simulink model "TRN_current"  (Simulink 6.2)
settings: Solver=ode45  SolverMode=SingleTasking  StartTime=0  StopTime=6  MaxStep=0.1  RelTol=1e-3  AbsTol=1e-3
libraries: simulink x1
(part 2 of 3)

== system TRN_current/Basal Ganglia/Striatum(D1)/chan1 ==
  note: Dopamine
      | modulation
  dopamine : Inport  Orientation=down  Port=1  PortDimensions=1  LatchInput=off
  cortex : Inport  Orientation=down  Port=2  LatchInput=off
  salience : Inport  Orientation=down  Port=3  LatchInput=off
  Constant : Constant  Orientation=down
  Product : Product  Orientation=down  SaturateOnIntegerOverflow=on  RndMeth=Zero  InputSameDT=on
  Sum : Sum  Orientation=down  SaturateOnIntegerOverflow=on  InputSameDT=on
  Sum1 : Sum  Orientation=down  SaturateOnIntegerOverflow=on  InputSameDT=on
  leaky integration : Subsystem  Orientation=down
  piecewise lin. : S-Function  Orientation=down  FunctionName=Mpieclin  Parameters=slope,thresh
  weight : Gain  Orientation=down  Gain=W_ctx  SaturateOnIntegerOverflow=on
  weight1 : Gain  Orientation=down  Gain=W_sal  SaturateOnIntegerOverflow=on
  out : Outport  Orientation=down  InitialOutput=0
  wires:
  Product/1 -> leaky integration/1(Inport)
  Constant/1 -> Sum/1
  piecewise lin./1 -> out/1
  leaky integration/1(Outport) -> piecewise lin./1
  dopamine/1 -> Sum/2
  Sum/1 -> Product/1
  cortex/1 -> weight/1
  salience/1 -> weight1/1
  weight/1 -> Sum1/1
  weight1/1 -> Sum1/2
  Sum1/1 -> Product/2

== system TRN_current/Basal Ganglia/Striatum(D1)/chan2 ==
  note: Dopamine
      | modulation
  dopamine : Inport  Orientation=down  Port=1  PortDimensions=1  LatchInput=off
  cortex : Inport  Orientation=down  Port=2  LatchInput=off
  salience : Inport  Orientation=down  Port=3  LatchInput=off
  Constant : Constant  Orientation=down
  Product : Product  Orientation=down  SaturateOnIntegerOverflow=on  RndMeth=Zero  InputSameDT=on
  Sum : Sum  Orientation=down  SaturateOnIntegerOverflow=on  InputSameDT=on
  Sum1 : Sum  Orientation=down  SaturateOnIntegerOverflow=on  InputSameDT=on
  leaky integration : Subsystem  Orientation=down
  piecewise lin. : S-Function  Orientation=down  FunctionName=Mpieclin  Parameters=slope,thresh
  weight : Gain  Orientation=down  Gain=W_ctx  SaturateOnIntegerOverflow=on
  weight1 : Gain  Orientation=down  Gain=W_sal  SaturateOnIntegerOverflow=on
  out : Outport  Orientation=down  InitialOutput=0
  wires:
  Sum1/1 -> Product/2
  weight1/1 -> Sum1/2
  weight/1 -> Sum1/1
  salience/1 -> weight1/1
  cortex/1 -> weight/1
  Sum/1 -> Product/1
  dopamine/1 -> Sum/2
  leaky integration/1(Outport) -> piecewise lin./1
  piecewise lin./1 -> out/1
  Constant/1 -> Sum/1
  Product/1 -> leaky integration/1(Inport)

== system TRN_current/Basal Ganglia/Striatum(D1)/chan3 ==
  note: Dopamine
      | modulation
  dopamine : Inport  Orientation=down  Port=1  PortDimensions=1  LatchInput=off
  cortex : Inport  Orientation=down  Port=2  LatchInput=off
  salience : Inport  Orientation=down  Port=3  LatchInput=off
  Constant : Constant  Orientation=down
  Product : Product  Orientation=down  SaturateOnIntegerOverflow=on  RndMeth=Zero  InputSameDT=on
  Sum : Sum  Orientation=down  SaturateOnIntegerOverflow=on  InputSameDT=on
  Sum1 : Sum  Orientation=down  SaturateOnIntegerOverflow=on  InputSameDT=on
  leaky integration : Subsystem  Orientation=down
  piecewise lin. : S-Function  Orientation=down  FunctionName=Mpieclin  Parameters=slope,thresh
  weight : Gain  Orientation=down  Gain=W_ctx  SaturateOnIntegerOverflow=on
  weight1 : Gain  Orientation=down  Gain=W_sal  SaturateOnIntegerOverflow=on
  out : Outport  Orientation=down  InitialOutput=0
  wires:
  Product/1 -> leaky integration/1(Inport)
  Constant/1 -> Sum/1
  piecewise lin./1 -> out/1
  leaky integration/1(Outport) -> piecewise lin./1
  dopamine/1 -> Sum/2
  Sum/1 -> Product/1
  cortex/1 -> weight/1
  salience/1 -> weight1/1
  weight/1 -> Sum1/1
  weight1/1 -> Sum1/2
  Sum1/1 -> Product/2

== system TRN_current/Basal Ganglia/Striatum(D1)/chan4 ==
  note: Dopamine
      | modulation
  dopamine : Inport  Orientation=down  Port=1  PortDimensions=1  LatchInput=off
  cortex : Inport  Orientation=down  Port=2  LatchInput=off
  salience : Inport  Orientation=down  Port=3  LatchInput=off
  Constant : Constant  Orientation=down
  Product : Product  Orientation=down  SaturateOnIntegerOverflow=on  RndMeth=Zero  InputSameDT=on
  Sum : Sum  Orientation=down  SaturateOnIntegerOverflow=on  InputSameDT=on
  Sum1 : Sum  Orientation=down  SaturateOnIntegerOverflow=on  InputSameDT=on
  leaky integration : Subsystem  Orientation=down
  piecewise lin. : S-Function  Orientation=down  FunctionName=Mpieclin  Parameters=slope,thresh
  weight : Gain  Orientation=down  Gain=W_ctx  SaturateOnIntegerOverflow=on
  weight1 : Gain  Orientation=down  Gain=W_sal  SaturateOnIntegerOverflow=on
  out : Outport  Orientation=down  InitialOutput=0
  wires:
  Sum1/1 -> Product/2
  weight1/1 -> Sum1/2
  weight/1 -> Sum1/1
  salience/1 -> weight1/1
  cortex/1 -> weight/1
  Sum/1 -> Product/1
  dopamine/1 -> Sum/2
  leaky integration/1(Outport) -> piecewise lin./1
  piecewise lin./1 -> out/1
  Constant/1 -> Sum/1
  Product/1 -> leaky integration/1(Inport)

== system TRN_current/Basal Ganglia/Striatum(D1)/chan5 ==
  note: Dopamine
      | modulation
  dopamine : Inport  Orientation=down  Port=1  PortDimensions=1  LatchInput=off
  cortex : Inport  Orientation=down  Port=2  LatchInput=off
  salience : Inport  Orientation=down  Port=3  LatchInput=off
  Constant : Constant  Orientation=down
  Product : Product  Orientation=down  SaturateOnIntegerOverflow=on  RndMeth=Zero  InputSameDT=on
  Sum : Sum  Orientation=down  SaturateOnIntegerOverflow=on  InputSameDT=on
  Sum1 : Sum  Orientation=down  SaturateOnIntegerOverflow=on  InputSameDT=on
  leaky integration : Subsystem  Orientation=down
  piecewise lin. : S-Function  Orientation=down  FunctionName=Mpieclin  Parameters=slope,thresh
  weight : Gain  Orientation=down  Gain=W_ctx  SaturateOnIntegerOverflow=on
  weight1 : Gain  Orientation=down  Gain=W_sal  SaturateOnIntegerOverflow=on
  out : Outport  Orientation=down  InitialOutput=0
  wires:
  Product/1 -> leaky integration/1(Inport)
  Constant/1 -> Sum/1
  piecewise lin./1 -> out/1
  leaky integration/1(Outport) -> piecewise lin./1
  dopamine/1 -> Sum/2
  Sum/1 -> Product/1
  cortex/1 -> weight/1
  salience/1 -> weight1/1
  weight/1 -> Sum1/1
  weight1/1 -> Sum1/2
  Sum1/1 -> Product/2

== system TRN_current/Basal Ganglia/Striatum(D1)/chan6 ==
  note: Dopamine
      | modulation
  dopamine : Inport  Orientation=down  Port=1  PortDimensions=1  LatchInput=off
  cortex : Inport  Orientation=down  Port=2  LatchInput=off
  salience : Inport  Orientation=down  Port=3  LatchInput=off
  Constant : Constant  Orientation=down
  Product : Product  Orientation=down  SaturateOnIntegerOverflow=on  RndMeth=Zero  InputSameDT=on
  Sum : Sum  Orientation=down  SaturateOnIntegerOverflow=on  InputSameDT=on
  Sum1 : Sum  Orientation=down  SaturateOnIntegerOverflow=on  InputSameDT=on
  leaky integration : Subsystem  Orientation=down
  piecewise lin. : S-Function  Orientation=down  FunctionName=Mpieclin  Parameters=slope,thresh
  weight : Gain  Orientation=down  Gain=W_ctx  SaturateOnIntegerOverflow=on
  weight1 : Gain  Orientation=down  Gain=W_sal  SaturateOnIntegerOverflow=on
  out : Outport  Orientation=down  InitialOutput=0
  wires:
  Sum1/1 -> Product/2
  weight1/1 -> Sum1/2
  weight/1 -> Sum1/1
  salience/1 -> weight1/1
  cortex/1 -> weight/1
  Sum/1 -> Product/1
  dopamine/1 -> Sum/2
  leaky integration/1(Outport) -> piecewise lin./1
  piecewise lin./1 -> out/1
  Constant/1 -> Sum/1
  Product/1 -> leaky integration/1(Inport)

== system TRN_current/Basal Ganglia/Striatum(D2)/chan1 ==
  note: Dopamine
      | modulation
  dopamine : Inport  Orientation=down  Port=1  PortDimensions=1  LatchInput=off
  cortex : Inport  Orientation=down  Port=2  LatchInput=off
  salience : Inport  Orientation=down  Port=3  LatchInput=off
  Constant : Constant  Orientation=down
  Product : Product  Orientation=down  SaturateOnIntegerOverflow=on  RndMeth=Zero  InputSameDT=on
  Sum : Sum  Orientation=down  Inputs=+-  SaturateOnIntegerOverflow=on  InputSameDT=on
  Sum1 : Sum  Orientation=down  SaturateOnIntegerOverflow=on  InputSameDT=on
  leaky integration : Subsystem  Orientation=down
  piecewise lin. : S-Function  Orientation=down  FunctionName=Mpieclin  Parameters=slope,thresh
  weight : Gain  Orientation=down  Gain=W_ctx  SaturateOnIntegerOverflow=on
  weight1 : Gain  Orientation=down  Gain=W_sal  SaturateOnIntegerOverflow=on
  out : Outport  Orientation=down  InitialOutput=0
  wires:
  Sum1/1 -> Product/2
  weight1/1 -> Sum1/2
  weight/1 -> Sum1/1
  salience/1 -> weight1/1
  cortex/1 -> weight/1
  Sum/1 -> Product/1
  dopamine/1 -> Sum/2
  leaky integration/1(Outport) -> piecewise lin./1
  piecewise lin./1 -> out/1
  Constant/1 -> Sum/1
  Product/1 -> leaky integration/1(Inport)

== system TRN_current/Basal Ganglia/Striatum(D2)/chan2 ==
  note: Dopamine
      | modulation
  dopamine : Inport  Orientation=down  Port=1  PortDimensions=1  LatchInput=off
  cortex : Inport  Orientation=down  Port=2  LatchInput=off
  salience : Inport  Orientation=down  Port=3  LatchInput=off
  Constant : Constant  Orientation=down
  Product : Product  Orientation=down  SaturateOnIntegerOverflow=on  RndMeth=Zero  InputSameDT=on
  Sum : Sum  Orientation=down  Inputs=+-  SaturateOnIntegerOverflow=on  InputSameDT=on
  Sum1 : Sum  Orientation=down  SaturateOnIntegerOverflow=on  InputSameDT=on
  leaky integration : Subsystem  Orientation=down
  piecewise lin. : S-Function  Orientation=down  FunctionName=Mpieclin  Parameters=slope,thresh
  weight : Gain  Orientation=down  Gain=W_ctx  SaturateOnIntegerOverflow=on
  weight1 : Gain  Orientation=down  Gain=W_sal  SaturateOnIntegerOverflow=on
  out : Outport  Orientation=down  InitialOutput=0
  wires:
  Product/1 -> leaky integration/1(Inport)
  Constant/1 -> Sum/1
  piecewise lin./1 -> out/1
  leaky integration/1(Outport) -> piecewise lin./1
  dopamine/1 -> Sum/2
  Sum/1 -> Product/1
  cortex/1 -> weight/1
  salience/1 -> weight1/1
  weight/1 -> Sum1/1
  weight1/1 -> Sum1/2
  Sum1/1 -> Product/2

== system TRN_current/Basal Ganglia/Striatum(D2)/chan3 ==
  note: Dopamine
      | modulation
  dopamine : Inport  Orientation=down  Port=1  PortDimensions=1  LatchInput=off
  cortex : Inport  Orientation=down  Port=2  LatchInput=off
  salience : Inport  Orientation=down  Port=3  LatchInput=off
  Constant : Constant  Orientation=down
  Product : Product  Orientation=down  SaturateOnIntegerOverflow=on  RndMeth=Zero  InputSameDT=on
  Sum : Sum  Orientation=down  Inputs=+-  SaturateOnIntegerOverflow=on  InputSameDT=on
  Sum1 : Sum  Orientation=down  SaturateOnIntegerOverflow=on  InputSameDT=on
  leaky integration : Subsystem  Orientation=down
  piecewise lin. : S-Function  Orientation=down  FunctionName=Mpieclin  Parameters=slope,thresh
  weight : Gain  Orientation=down  Gain=W_ctx  SaturateOnIntegerOverflow=on
  weight1 : Gain  Orientation=down  Gain=W_sal  SaturateOnIntegerOverflow=on
  out : Outport  Orientation=down  InitialOutput=0
  wires:
  Sum1/1 -> Product/2
  weight1/1 -> Sum1/2
  weight/1 -> Sum1/1
  salience/1 -> weight1/1
  cortex/1 -> weight/1
  Sum/1 -> Product/1
  dopamine/1 -> Sum/2
  leaky integration/1(Outport) -> piecewise lin./1
  piecewise lin./1 -> out/1
  Constant/1 -> Sum/1
  Product/1 -> leaky integration/1(Inport)

== system TRN_current/Basal Ganglia/Striatum(D2)/chan4 ==
  note: Dopamine
      | modulation
  dopamine : Inport  Orientation=down  Port=1  PortDimensions=1  LatchInput=off
  cortex : Inport  Orientation=down  Port=2  LatchInput=off
  salience : Inport  Orientation=down  Port=3  LatchInput=off
  Constant : Constant  Orientation=down
  Product : Product  Orientation=down  SaturateOnIntegerOverflow=on  RndMeth=Zero  InputSameDT=on
  Sum : Sum  Orientation=down  Inputs=+-  SaturateOnIntegerOverflow=on  InputSameDT=on
  Sum1 : Sum  Orientation=down  SaturateOnIntegerOverflow=on  InputSameDT=on
  leaky integration : Subsystem  Orientation=down
  piecewise lin. : S-Function  Orientation=down  FunctionName=Mpieclin  Parameters=slope,thresh
  weight : Gain  Orientation=down  Gain=W_ctx  SaturateOnIntegerOverflow=on
  weight1 : Gain  Orientation=down  Gain=W_sal  SaturateOnIntegerOverflow=on
  out : Outport  Orientation=down  InitialOutput=0
  wires:
  Product/1 -> leaky integration/1(Inport)
  Constant/1 -> Sum/1
  piecewise lin./1 -> out/1
  leaky integration/1(Outport) -> piecewise lin./1
  dopamine/1 -> Sum/2
  Sum/1 -> Product/1
  cortex/1 -> weight/1
  salience/1 -> weight1/1
  weight/1 -> Sum1/1
  weight1/1 -> Sum1/2
  Sum1/1 -> Product/2

== system TRN_current/Basal Ganglia/Striatum(D2)/chan5 ==
  note: Dopamine
      | modulation
  dopamine : Inport  Orientation=down  Port=1  PortDimensions=1  LatchInput=off
  cortex : Inport  Orientation=down  Port=2  LatchInput=off
  salience : Inport  Orientation=down  Port=3  LatchInput=off
  Constant : Constant  Orientation=down
  Product : Product  Orientation=down  SaturateOnIntegerOverflow=on  RndMeth=Zero  InputSameDT=on
  Sum : Sum  Orientation=down  Inputs=+-  SaturateOnIntegerOverflow=on  InputSameDT=on
  Sum1 : Sum  Orientation=down  SaturateOnIntegerOverflow=on  InputSameDT=on
  leaky integration : Subsystem  Orientation=down
  piecewise lin. : S-Function  Orientation=down  FunctionName=Mpieclin  Parameters=slope,thresh
  weight : Gain  Orientation=down  Gain=W_ctx  SaturateOnIntegerOverflow=on
  weight1 : Gain  Orientation=down  Gain=W_sal  SaturateOnIntegerOverflow=on
  out : Outport  Orientation=down  InitialOutput=0
  wires:
  Sum1/1 -> Product/2
  weight1/1 -> Sum1/2
  weight/1 -> Sum1/1
  salience/1 -> weight1/1
  cortex/1 -> weight/1
  Sum/1 -> Product/1
  dopamine/1 -> Sum/2
  leaky integration/1(Outport) -> piecewise lin./1
  piecewise lin./1 -> out/1
  Constant/1 -> Sum/1
  Product/1 -> leaky integration/1(Inport)

== system TRN_current/Basal Ganglia/Striatum(D2)/chan6 ==
  note: Dopamine
      | modulation
  dopamine : Inport  Orientation=down  Port=1  PortDimensions=1  LatchInput=off
  cortex : Inport  Orientation=down  Port=2  LatchInput=off
  salience : Inport  Orientation=down  Port=3  LatchInput=off
  Constant : Constant  Orientation=down
  Product : Product  Orientation=down  SaturateOnIntegerOverflow=on  RndMeth=Zero  InputSameDT=on
  Sum : Sum  Orientation=down  Inputs=+-  SaturateOnIntegerOverflow=on  InputSameDT=on
  Sum1 : Sum  Orientation=down  SaturateOnIntegerOverflow=on  InputSameDT=on
  leaky integration : Subsystem  Orientation=down
  piecewise lin. : S-Function  Orientation=down  FunctionName=Mpieclin  Parameters=slope,thresh
  weight : Gain  Orientation=down  Gain=W_ctx  SaturateOnIntegerOverflow=on
  weight1 : Gain  Orientation=down  Gain=W_sal  SaturateOnIntegerOverflow=on
  out : Outport  Orientation=down  InitialOutput=0
  wires:
  Product/1 -> leaky integration/1(Inport)
  Constant/1 -> Sum/1
  piecewise lin./1 -> out/1
  leaky integration/1(Outport) -> piecewise lin./1
  dopamine/1 -> Sum/2
  Sum/1 -> Product/1
  cortex/1 -> weight/1
  salience/1 -> weight1/1
  weight/1 -> Sum1/1
  weight1/1 -> Sum1/2
  Sum1/1 -> Product/2

== system TRN_current/Motor  Cortex/chan1/leaky integration ==
  Inport : Inport  Port=1  PortDimensions=1  LatchInput=off
  Gain : Gain  Gain=A_rate  SaturateOnIntegerOverflow=on
  Integrator : Integrator
  decay const : Gain  Orientation=left  Gain=-A_rate  SaturateOnIntegerOverflow=on
  sum : Sum  SaturateOnIntegerOverflow=on  InputSameDT=on
  Outport : Outport  InitialOutput=0
  wires:
  decay const/1 -> sum/2
  sum/1 -> Integrator/1
  Integrator/1 -> decay const/1, Outport/1
  Inport/1 -> Gain/1
  Gain/1 -> sum/1

== system TRN_current/Motor  Cortex/chan2/leaky integration ==
  Inport : Inport  Port=1  PortDimensions=1  LatchInput=off
  Gain : Gain  Gain=A_rate  SaturateOnIntegerOverflow=on
  Integrator : Integrator
  decay const : Gain  Orientation=left  Gain=-A_rate  SaturateOnIntegerOverflow=on
  sum : Sum  SaturateOnIntegerOverflow=on  InputSameDT=on
  Outport : Outport  InitialOutput=0
  wires:
  Gain/1 -> sum/1
  Inport/1 -> Gain/1
  Integrator/1 -> Outport/1, decay const/1
  sum/1 -> Integrator/1
  decay const/1 -> sum/2

== system TRN_current/Motor  Cortex/chan3/leaky integration ==
  Inport : Inport  Port=1  PortDimensions=1  LatchInput=off
  Gain : Gain  Gain=A_rate  SaturateOnIntegerOverflow=on
  Integrator : Integrator
  decay const : Gain  Orientation=left  Gain=-A_rate  SaturateOnIntegerOverflow=on
  sum : Sum  SaturateOnIntegerOverflow=on  InputSameDT=on
  Outport : Outport  InitialOutput=0
  wires:
  decay const/1 -> sum/2
  sum/1 -> Integrator/1
  Integrator/1 -> decay const/1, Outport/1
  Inport/1 -> Gain/1
  Gain/1 -> sum/1

== system TRN_current/Motor  Cortex/chan4/leaky integration ==
  Inport : Inport  Port=1  PortDimensions=1  LatchInput=off
  Gain : Gain  Gain=A_rate  SaturateOnIntegerOverflow=on
  Integrator : Integrator
  decay const : Gain  Orientation=left  Gain=-A_rate  SaturateOnIntegerOverflow=on
  sum : Sum  SaturateOnIntegerOverflow=on  InputSameDT=on
  Outport : Outport  InitialOutput=0
  wires:
  Gain/1 -> sum/1
  Inport/1 -> Gain/1
  Integrator/1 -> Outport/1, decay const/1
  sum/1 -> Integrator/1
  decay const/1 -> sum/2

== system TRN_current/Motor  Cortex/chan5/leaky integration ==
  Inport : Inport  Port=1  PortDimensions=1  LatchInput=off
  Gain : Gain  Gain=A_rate  SaturateOnIntegerOverflow=on
  Integrator : Integrator
  decay const : Gain  Orientation=left  Gain=-A_rate  SaturateOnIntegerOverflow=on
  sum : Sum  SaturateOnIntegerOverflow=on  InputSameDT=on
  Outport : Outport  InitialOutput=0
  wires:
  decay const/1 -> sum/2
  sum/1 -> Integrator/1
  Integrator/1 -> decay const/1, Outport/1
  Inport/1 -> Gain/1
  Gain/1 -> sum/1

== system TRN_current/Motor  Cortex/chan6/leaky integration ==
  Inport : Inport  Port=1  PortDimensions=1  LatchInput=off
  Gain : Gain  Gain=A_rate  SaturateOnIntegerOverflow=on
  Integrator : Integrator
  decay const : Gain  Orientation=left  Gain=-A_rate  SaturateOnIntegerOverflow=on
  sum : Sum  SaturateOnIntegerOverflow=on  InputSameDT=on
  Outport : Outport  InitialOutput=0
  wires:
  Gain/1 -> sum/1
  Inport/1 -> Gain/1
  Integrator/1 -> Outport/1, decay const/1
  sum/1 -> Integrator/1
  decay const/1 -> sum/2

== system TRN_current/TRN/chan1/leaky integration ==
  Inport : Inport  Port=1  PortDimensions=1  LatchInput=off
  Gain : Gain  Gain=A_rate  SaturateOnIntegerOverflow=on
  Integrator : Integrator
  decay const : Gain  Orientation=left  Gain=-A_rate  SaturateOnIntegerOverflow=on
  sum : Sum  SaturateOnIntegerOverflow=on  InputSameDT=on
  Outport : Outport  InitialOutput=0
  wires:
  decay const/1 -> sum/2
  sum/1 -> Integrator/1
  Integrator/1 -> decay const/1, Outport/1
  Inport/1 -> Gain/1
  Gain/1 -> sum/1

== system TRN_current/TRN/chan2/leaky integration ==
  Inport : Inport  Port=1  PortDimensions=1  LatchInput=off
  Gain : Gain  Gain=A_rate  SaturateOnIntegerOverflow=on
  Integrator : Integrator
  decay const : Gain  Orientation=left  Gain=-A_rate  SaturateOnIntegerOverflow=on
  sum : Sum  SaturateOnIntegerOverflow=on  InputSameDT=on
  Outport : Outport  InitialOutput=0
  wires:
  Gain/1 -> sum/1
  Inport/1 -> Gain/1
  Integrator/1 -> Outport/1, decay const/1
  sum/1 -> Integrator/1
  decay const/1 -> sum/2

== system TRN_current/TRN/chan3/leaky integration ==
  Inport : Inport  Port=1  PortDimensions=1  LatchInput=off
  Gain : Gain  Gain=A_rate  SaturateOnIntegerOverflow=on
  Integrator : Integrator
  decay const : Gain  Orientation=left  Gain=-A_rate  SaturateOnIntegerOverflow=on
  sum : Sum  SaturateOnIntegerOverflow=on  InputSameDT=on
  Outport : Outport  InitialOutput=0
  wires:
  decay const/1 -> sum/2
  sum/1 -> Integrator/1
  Integrator/1 -> decay const/1, Outport/1
  Inport/1 -> Gain/1
  Gain/1 -> sum/1

== system TRN_current/TRN/chan4/leaky integration ==
  Inport : Inport  Port=1  PortDimensions=1  LatchInput=off
  Gain : Gain  Gain=A_rate  SaturateOnIntegerOverflow=on
  Integrator : Integrator
  decay const : Gain  Orientation=left  Gain=-A_rate  SaturateOnIntegerOverflow=on
  sum : Sum  SaturateOnIntegerOverflow=on  InputSameDT=on
  Outport : Outport  InitialOutput=0
  wires:
  Gain/1 -> sum/1
  Inport/1 -> Gain/1
  Integrator/1 -> Outport/1, decay const/1
  sum/1 -> Integrator/1
  decay const/1 -> sum/2

== system TRN_current/TRN/chan5/leaky integration ==
  Inport : Inport  Port=1  PortDimensions=1  LatchInput=off
  Gain : Gain  Gain=A_rate  SaturateOnIntegerOverflow=on
  Integrator : Integrator
  decay const : Gain  Orientation=left  Gain=-A_rate  SaturateOnIntegerOverflow=on
  sum : Sum  SaturateOnIntegerOverflow=on  InputSameDT=on
  Outport : Outport  InitialOutput=0
  wires:
  decay const/1 -> sum/2
  sum/1 -> Integrator/1
  Integrator/1 -> decay const/1, Outport/1
  Inport/1 -> Gain/1
  Gain/1 -> sum/1

== system TRN_current/TRN/chan6/leaky integration ==
  Inport : Inport  Port=1  PortDimensions=1  LatchInput=off
  Gain : Gain  Gain=A_rate  SaturateOnIntegerOverflow=on
  Integrator : Integrator
  decay const : Gain  Orientation=left  Gain=-A_rate  SaturateOnIntegerOverflow=on
  sum : Sum  SaturateOnIntegerOverflow=on  InputSameDT=on
  Outport : Outport  InitialOutput=0
  wires:
  Gain/1 -> sum/1
  Inport/1 -> Gain/1
  Integrator/1 -> Outport/1, decay const/1
  sum/1 -> Integrator/1
  decay const/1 -> sum/2

== system TRN_current/Ventrolateral Thalamus/chan1/leaky integration ==
  Inport : Inport  Port=1  PortDimensions=1  LatchInput=off
  Gain : Gain  Gain=A_rate  SaturateOnIntegerOverflow=on
  Integrator : Integrator
  decay const : Gain  Orientation=left  Gain=-A_rate  SaturateOnIntegerOverflow=on
  sum : Sum  SaturateOnIntegerOverflow=on  InputSameDT=on
  Outport : Outport  InitialOutput=0
  wires:
  decay const/1 -> sum/2
  sum/1 -> Integrator/1
  Integrator/1 -> decay const/1, Outport/1
  Inport/1 -> Gain/1
  Gain/1 -> sum/1

== system TRN_current/Ventrolateral Thalamus/chan2/leaky integration ==
  Inport : Inport  Port=1  PortDimensions=1  LatchInput=off
  Gain : Gain  Gain=A_rate  SaturateOnIntegerOverflow=on
  Integrator : Integrator
  decay const : Gain  Orientation=left  Gain=-A_rate  SaturateOnIntegerOverflow=on
  sum : Sum  SaturateOnIntegerOverflow=on  InputSameDT=on
  Outport : Outport  InitialOutput=0
  wires:
  Gain/1 -> sum/1
  Inport/1 -> Gain/1
  Integrator/1 -> Outport/1, decay const/1
  sum/1 -> Integrator/1
  decay const/1 -> sum/2

== system TRN_current/Ventrolateral Thalamus/chan3/leaky integration ==
  Inport : Inport  Port=1  PortDimensions=1  LatchInput=off
  Gain : Gain  Gain=A_rate  SaturateOnIntegerOverflow=on
  Integrator : Integrator
  decay const : Gain  Orientation=left  Gain=-A_rate  SaturateOnIntegerOverflow=on
  sum : Sum  SaturateOnIntegerOverflow=on  InputSameDT=on
  Outport : Outport  InitialOutput=0
  wires:
  decay const/1 -> sum/2
  sum/1 -> Integrator/1
  Integrator/1 -> decay const/1, Outport/1
  Inport/1 -> Gain/1
  Gain/1 -> sum/1

== system TRN_current/Ventrolateral Thalamus/chan4/leaky integration ==
  Inport : Inport  Port=1  PortDimensions=1  LatchInput=off
  Gain : Gain  Gain=A_rate  SaturateOnIntegerOverflow=on
  Integrator : Integrator
  decay const : Gain  Orientation=left  Gain=-A_rate  SaturateOnIntegerOverflow=on
  sum : Sum  SaturateOnIntegerOverflow=on  InputSameDT=on
  Outport : Outport  InitialOutput=0
  wires:
  Gain/1 -> sum/1
  Inport/1 -> Gain/1
  Integrator/1 -> Outport/1, decay const/1
  sum/1 -> Integrator/1
  decay const/1 -> sum/2

== system TRN_current/Ventrolateral Thalamus/chan5/leaky integration ==
  Inport : Inport  Port=1  PortDimensions=1  LatchInput=off
  Gain : Gain  Gain=A_rate  SaturateOnIntegerOverflow=on
  Integrator : Integrator
  decay const : Gain  Orientation=left  Gain=-A_rate  SaturateOnIntegerOverflow=on
  sum : Sum  SaturateOnIntegerOverflow=on  InputSameDT=on
  Outport : Outport  InitialOutput=0
  wires:
  decay const/1 -> sum/2
  sum/1 -> Integrator/1
  Integrator/1 -> decay const/1, Outport/1
  Inport/1 -> Gain/1
  Gain/1 -> sum/1

== system TRN_current/Ventrolateral Thalamus/chan6/leaky integration ==
  Inport : Inport  Port=1  PortDimensions=1  LatchInput=off
  Gain : Gain  Gain=A_rate  SaturateOnIntegerOverflow=on
  Integrator : Integrator
  decay const : Gain  Orientation=left  Gain=-A_rate  SaturateOnIntegerOverflow=on
  sum : Sum  SaturateOnIntegerOverflow=on  InputSameDT=on
  Outport : Outport  InitialOutput=0
  wires:
  Gain/1 -> sum/1
  Inport/1 -> Gain/1
  Integrator/1 -> Outport/1, decay const/1
  sum/1 -> Integrator/1
  decay const/1 -> sum/2

== system TRN_current/Basal Ganglia/GPe/2 input channel/input summation ==
  x1 : Inport  Port=1  LatchInput=off
  x2 : Inport  Port=2  LatchInput=off
  Sum : Sum  SaturateOnIntegerOverflow=on  InputSameDT=on
  W1 : Gain  Gain=W_str  SaturateOnIntegerOverflow=on
  W2 : Gain  Gain=W_STN  SaturateOnIntegerOverflow=on
  out_1 : Outport  InitialOutput=0
  wires:
  W2/1 -> Sum/2
  W1/1 -> Sum/1
  x2/1 -> W2/1
  x1/1 -> W1/1
  Sum/1 -> out_1/1

== system TRN_current/Basal Ganglia/GPe/2 input channel/leaky integration ==
  Inport : Inport  Port=1  LatchInput=off
  Gain : Gain  Gain=A_rate  SaturateOnIntegerOverflow=on
  Integrator : Integrator
  decay const : Gain  Orientation=left  Gain=-A_rate  SaturateOnIntegerOverflow=on
  sum : Sum  SaturateOnIntegerOverflow=on  InputSameDT=on
  Outport : Outport  InitialOutput=0
  wires:
  Gain/1 -> sum/1
  Inport/1 -> Gain/1
  Integrator/1 -> decay const/1, Outport/1
  sum/1 -> Integrator/1
  decay const/1 -> sum/2

== system TRN_current/Basal Ganglia/GPe/2 input channel1/input summation ==
  x1 : Inport  Port=1  LatchInput=off
  x2 : Inport  Port=2  LatchInput=off
  Sum : Sum  SaturateOnIntegerOverflow=on  InputSameDT=on
  W1 : Gain  Gain=W_str  SaturateOnIntegerOverflow=on
  W2 : Gain  Gain=W_STN  SaturateOnIntegerOverflow=on
  out_1 : Outport  InitialOutput=0
  wires:
  Sum/1 -> out_1/1
  x1/1 -> W1/1
  x2/1 -> W2/1
  W1/1 -> Sum/1
  W2/1 -> Sum/2

== system TRN_current/Basal Ganglia/GPe/2 input channel1/leaky integration ==
  Inport : Inport  Port=1  LatchInput=off
  Gain : Gain  Gain=A_rate  SaturateOnIntegerOverflow=on
  Integrator : Integrator
  decay const : Gain  Orientation=left  Gain=-A_rate  SaturateOnIntegerOverflow=on
  sum : Sum  SaturateOnIntegerOverflow=on  InputSameDT=on
  Outport : Outport  InitialOutput=0
  wires:
  decay const/1 -> sum/2
  sum/1 -> Integrator/1
  Integrator/1 -> Outport/1, decay const/1
  Inport/1 -> Gain/1
  Gain/1 -> sum/1

== system TRN_current/Basal Ganglia/GPe/2 input channel2/input summation ==
  x1 : Inport  Port=1  LatchInput=off
  x2 : Inport  Port=2  LatchInput=off
  Sum : Sum  SaturateOnIntegerOverflow=on  InputSameDT=on
  W1 : Gain  Gain=W_str  SaturateOnIntegerOverflow=on
  W2 : Gain  Gain=W_STN  SaturateOnIntegerOverflow=on
  out_1 : Outport  InitialOutput=0
  wires:
  W2/1 -> Sum/2
  W1/1 -> Sum/1
  x2/1 -> W2/1
  x1/1 -> W1/1
  Sum/1 -> out_1/1

== system TRN_current/Basal Ganglia/GPe/2 input channel2/leaky integration ==
  Inport : Inport  Port=1  LatchInput=off
  Gain : Gain  Gain=A_rate  SaturateOnIntegerOverflow=on
  Integrator : Integrator
  decay const : Gain  Orientation=left  Gain=-A_rate  SaturateOnIntegerOverflow=on
  sum : Sum  SaturateOnIntegerOverflow=on  InputSameDT=on
  Outport : Outport  InitialOutput=0
  wires:
  Gain/1 -> sum/1
  Inport/1 -> Gain/1
  Integrator/1 -> decay const/1, Outport/1
  sum/1 -> Integrator/1
  decay const/1 -> sum/2

== system TRN_current/Basal Ganglia/GPe/2 input channel3/input summation ==
  x1 : Inport  Port=1  LatchInput=off
  x2 : Inport  Port=2  LatchInput=off
  Sum : Sum  SaturateOnIntegerOverflow=on  InputSameDT=on
  W1 : Gain  Gain=W_str  SaturateOnIntegerOverflow=on
  W2 : Gain  Gain=W_STN  SaturateOnIntegerOverflow=on
  out_1 : Outport  InitialOutput=0
  wires:
  Sum/1 -> out_1/1
  x1/1 -> W1/1
  x2/1 -> W2/1
  W1/1 -> Sum/1
  W2/1 -> Sum/2

== system TRN_current/Basal Ganglia/GPe/2 input channel3/leaky integration ==
  Inport : Inport  Port=1  LatchInput=off
  Gain : Gain  Gain=A_rate  SaturateOnIntegerOverflow=on
  Integrator : Integrator
  decay const : Gain  Orientation=left  Gain=-A_rate  SaturateOnIntegerOverflow=on
  sum : Sum  SaturateOnIntegerOverflow=on  InputSameDT=on
  Outport : Outport  InitialOutput=0
  wires:
  decay const/1 -> sum/2
  sum/1 -> Integrator/1
  Integrator/1 -> Outport/1, decay const/1
  Inport/1 -> Gain/1
  Gain/1 -> sum/1

== system TRN_current/Basal Ganglia/GPe/2 input channel4/input summation ==
  x1 : Inport  Port=1  LatchInput=off
  x2 : Inport  Port=2  LatchInput=off
  Sum : Sum  SaturateOnIntegerOverflow=on  InputSameDT=on
  W1 : Gain  Gain=W_str  SaturateOnIntegerOverflow=on
  W2 : Gain  Gain=W_STN  SaturateOnIntegerOverflow=on
  out_1 : Outport  InitialOutput=0
  wires:
  W2/1 -> Sum/2
  W1/1 -> Sum/1
  x2/1 -> W2/1
  x1/1 -> W1/1
  Sum/1 -> out_1/1

== system TRN_current/Basal Ganglia/GPe/2 input channel4/leaky integration ==
  Inport : Inport  Port=1  LatchInput=off
  Gain : Gain  Gain=A_rate  SaturateOnIntegerOverflow=on
  Integrator : Integrator
  decay const : Gain  Orientation=left  Gain=-A_rate  SaturateOnIntegerOverflow=on
  sum : Sum  SaturateOnIntegerOverflow=on  InputSameDT=on
  Outport : Outport  InitialOutput=0
  wires:
  Gain/1 -> sum/1
  Inport/1 -> Gain/1
  Integrator/1 -> decay const/1, Outport/1
  sum/1 -> Integrator/1
  decay const/1 -> sum/2

== system TRN_current/Basal Ganglia/GPe/2 input channel5/input summation ==
  x1 : Inport  Port=1  LatchInput=off
  x2 : Inport  Port=2  LatchInput=off
  Sum : Sum  SaturateOnIntegerOverflow=on  InputSameDT=on
  W1 : Gain  Gain=W_str  SaturateOnIntegerOverflow=on
  W2 : Gain  Gain=W_STN  SaturateOnIntegerOverflow=on
  out_1 : Outport  InitialOutput=0
  wires:
  Sum/1 -> out_1/1
  x1/1 -> W1/1
  x2/1 -> W2/1
  W1/1 -> Sum/1
  W2/1 -> Sum/2

== system TRN_current/Basal Ganglia/GPe/2 input channel5/leaky integration ==
  Inport : Inport  Port=1  LatchInput=off
  Gain : Gain  Gain=A_rate  SaturateOnIntegerOverflow=on
  Integrator : Integrator
  decay const : Gain  Orientation=left  Gain=-A_rate  SaturateOnIntegerOverflow=on
  sum : Sum  SaturateOnIntegerOverflow=on  InputSameDT=on
  Outport : Outport  InitialOutput=0
  wires:
  decay const/1 -> sum/2
  sum/1 -> Integrator/1
  Integrator/1 -> Outport/1, decay const/1
  Inport/1 -> Gain/1
  Gain/1 -> sum/1

== system TRN_current/Basal Ganglia/GPi/2 input channel/input summation ==
  x1 : Inport  Port=1  LatchInput=off
  x2 : Inport  Port=2  LatchInput=off
  x3 : Inport  Port=3  LatchInput=off
  Sum : Sum  Inputs=+++  SaturateOnIntegerOverflow=on  InputSameDT=on
  W1 : Gain  Gain=W_str  SaturateOnIntegerOverflow=on
  W2 : Gain  Gain=W_STN  SaturateOnIntegerOverflow=on
  W3 : Gain  Gain=W_GPe  SaturateOnIntegerOverflow=on
  out_1 : Outport  InitialOutput=0
  wires:
  Sum/1 -> out_1/1
  x1/1 -> W1/1
  x2/1 -> W2/1
  W1/1 -> Sum/1
  W2/1 -> Sum/2
  x3/1 -> W3/1
  W3/1 -> Sum/3

== system TRN_current/Basal Ganglia/GPi/2 input channel/leaky integration ==
  Inport : Inport  Port=1  LatchInput=off
  Gain : Gain  Gain=A_rate  SaturateOnIntegerOverflow=on
  Integrator : Integrator
  decay const : Gain  Orientation=left  Gain=-A_rate  SaturateOnIntegerOverflow=on
  sum : Sum  SaturateOnIntegerOverflow=on  InputSameDT=on
  Outport : Outport  InitialOutput=0
  wires:
  decay const/1 -> sum/2
  sum/1 -> Integrator/1
  Integrator/1 -> Outport/1, decay const/1
  Inport/1 -> Gain/1
  Gain/1 -> sum/1

== system TRN_current/Basal Ganglia/GPi/2 input channel1/input summation ==
  x1 : Inport  Port=1  LatchInput=off
  x2 : Inport  Port=2  LatchInput=off
  x3 : Inport  Port=3  LatchInput=off
  Sum : Sum  Inputs=+++  SaturateOnIntegerOverflow=on  InputSameDT=on
  W1 : Gain  Gain=W_str  SaturateOnIntegerOverflow=on
  W2 : Gain  Gain=W_STN  SaturateOnIntegerOverflow=on
  W3 : Gain  Gain=W_GPe  SaturateOnIntegerOverflow=on
  out_1 : Outport  InitialOutput=0
  wires:
  W3/1 -> Sum/3
  x3/1 -> W3/1
  W2/1 -> Sum/2
  W1/1 -> Sum/1
  x2/1 -> W2/1
  x1/1 -> W1/1
  Sum/1 -> out_1/1

== system TRN_current/Basal Ganglia/GPi/2 input channel1/leaky integration ==
  Inport : Inport  Port=1  LatchInput=off
  Gain : Gain  Gain=A_rate  SaturateOnIntegerOverflow=on
  Integrator : Integrator
  decay const : Gain  Orientation=left  Gain=-A_rate  SaturateOnIntegerOverflow=on
  sum : Sum  SaturateOnIntegerOverflow=on  InputSameDT=on
  Outport : Outport  InitialOutput=0
  wires:
  Gain/1 -> sum/1
  Inport/1 -> Gain/1
  Integrator/1 -> decay const/1, Outport/1
  sum/1 -> Integrator/1
  decay const/1 -> sum/2

== system TRN_current/Basal Ganglia/GPi/2 input channel2/input summation ==
  x1 : Inport  Port=1  LatchInput=off
  x2 : Inport  Port=2  LatchInput=off
  x3 : Inport  Port=3  LatchInput=off
  Sum : Sum  Inputs=+++  SaturateOnIntegerOverflow=on  InputSameDT=on
  W1 : Gain  Gain=W_str  SaturateOnIntegerOverflow=on
  W2 : Gain  Gain=W_STN  SaturateOnIntegerOverflow=on
  W3 : Gain  Gain=W_GPe  SaturateOnIntegerOverflow=on
  out_1 : Outport  InitialOutput=0
  wires:
  Sum/1 -> out_1/1
  x1/1 -> W1/1
  x2/1 -> W2/1
  W1/1 -> Sum/1
  W2/1 -> Sum/2
  x3/1 -> W3/1
  W3/1 -> Sum/3

== system TRN_current/Basal Ganglia/GPi/2 input channel2/leaky integration ==
  Inport : Inport  Port=1  LatchInput=off
  Gain : Gain  Gain=A_rate  SaturateOnIntegerOverflow=on
  Integrator : Integrator
  decay const : Gain  Orientation=left  Gain=-A_rate  SaturateOnIntegerOverflow=on
  sum : Sum  SaturateOnIntegerOverflow=on  InputSameDT=on
  Outport : Outport  InitialOutput=0
  wires:
  decay const/1 -> sum/2
  sum/1 -> Integrator/1
  Integrator/1 -> Outport/1, decay const/1
  Inport/1 -> Gain/1
  Gain/1 -> sum/1

== system TRN_current/Basal Ganglia/GPi/2 input channel3/input summation ==
  x1 : Inport  Port=1  LatchInput=off
  x2 : Inport  Port=2  LatchInput=off
  x3 : Inport  Port=3  LatchInput=off
  Sum : Sum  Inputs=+++  SaturateOnIntegerOverflow=on  InputSameDT=on
  W1 : Gain  Gain=W_str  SaturateOnIntegerOverflow=on
  W2 : Gain  Gain=W_STN  SaturateOnIntegerOverflow=on
  W3 : Gain  Gain=W_GPe  SaturateOnIntegerOverflow=on
  out_1 : Outport  InitialOutput=0
  wires:
  W3/1 -> Sum/3
  x3/1 -> W3/1
  W2/1 -> Sum/2
  W1/1 -> Sum/1
  x2/1 -> W2/1
  x1/1 -> W1/1
  Sum/1 -> out_1/1

== system TRN_current/Basal Ganglia/GPi/2 input channel3/leaky integration ==
  Inport : Inport  Port=1  LatchInput=off
  Gain : Gain  Gain=A_rate  SaturateOnIntegerOverflow=on
  Integrator : Integrator
  decay const : Gain  Orientation=left  Gain=-A_rate  SaturateOnIntegerOverflow=on
  sum : Sum  SaturateOnIntegerOverflow=on  InputSameDT=on
  Outport : Outport  InitialOutput=0
  wires:
  Gain/1 -> sum/1
  Inport/1 -> Gain/1
  Integrator/1 -> decay const/1, Outport/1
  sum/1 -> Integrator/1
  decay const/1 -> sum/2

== system TRN_current/Basal Ganglia/GPi/2 input channel4/input summation ==
  x1 : Inport  Port=1  LatchInput=off
  x2 : Inport  Port=2  LatchInput=off
  x3 : Inport  Port=3  LatchInput=off
  Sum : Sum  Inputs=+++  SaturateOnIntegerOverflow=on  InputSameDT=on
  W1 : Gain  Gain=W_str  SaturateOnIntegerOverflow=on
  W2 : Gain  Gain=W_STN  SaturateOnIntegerOverflow=on
  W3 : Gain  Gain=W_GPe  SaturateOnIntegerOverflow=on
  out_1 : Outport  InitialOutput=0
  wires:
  Sum/1 -> out_1/1
  x1/1 -> W1/1
  x2/1 -> W2/1
  W1/1 -> Sum/1
  W2/1 -> Sum/2
  x3/1 -> W3/1
  W3/1 -> Sum/3

== system TRN_current/Basal Ganglia/GPi/2 input channel4/leaky integration ==
  Inport : Inport  Port=1  LatchInput=off
  Gain : Gain  Gain=A_rate  SaturateOnIntegerOverflow=on
  Integrator : Integrator
  decay const : Gain  Orientation=left  Gain=-A_rate  SaturateOnIntegerOverflow=on
  sum : Sum  SaturateOnIntegerOverflow=on  InputSameDT=on
  Outport : Outport  InitialOutput=0
  wires:
  decay const/1 -> sum/2
  sum/1 -> Integrator/1
  Integrator/1 -> Outport/1, decay const/1
  Inport/1 -> Gain/1
  Gain/1 -> sum/1

== system TRN_current/Basal Ganglia/GPi/2 input channel5/input summation ==
  x1 : Inport  Port=1  LatchInput=off
  x2 : Inport  Port=2  LatchInput=off
  x3 : Inport  Port=3  LatchInput=off
  Sum : Sum  Inputs=+++  SaturateOnIntegerOverflow=on  InputSameDT=on
  W1 : Gain  Gain=W_str  SaturateOnIntegerOverflow=on
  W2 : Gain  Gain=W_STN  SaturateOnIntegerOverflow=on
  W3 : Gain  Gain=W_GPe  SaturateOnIntegerOverflow=on
  out_1 : Outport  InitialOutput=0
  wires:
  W3/1 -> Sum/3
  x3/1 -> W3/1
  W2/1 -> Sum/2
  W1/1 -> Sum/1
  x2/1 -> W2/1
  x1/1 -> W1/1
  Sum/1 -> out_1/1

== system TRN_current/Basal Ganglia/GPi/2 input channel5/leaky integration ==
  Inport : Inport  Port=1  LatchInput=off
  Gain : Gain  Gain=A_rate  SaturateOnIntegerOverflow=on
  Integrator : Integrator
  decay const : Gain  Orientation=left  Gain=-A_rate  SaturateOnIntegerOverflow=on
  sum : Sum  SaturateOnIntegerOverflow=on  InputSameDT=on
  Outport : Outport  InitialOutput=0
  wires:
  Gain/1 -> sum/1
  Inport/1 -> Gain/1
  Integrator/1 -> decay const/1, Outport/1
  sum/1 -> Integrator/1
  decay const/1 -> sum/2

== system TRN_current/Basal Ganglia/STN/STN discrete model/2 input channel ==
  Salience : Inport  Orientation=down  Port=1  LatchInput=off
  GPe : Inport  Orientation=down  Port=2  LatchInput=off
  Cortex : Inport  Orientation=down  Port=3  LatchInput=off
  input summation : Subsystem  Orientation=down
  leaky integration : Subsystem  Orientation=down
  piecewise lin. : S-Function  Orientation=down  FunctionName=Mpieclin  Parameters=slope,thresh
  out : Outport  Orientation=down  InitialOutput=0
  wires:
  piecewise lin./1 -> out/1
  GPe/1 -> input summation/2(x2)
  Salience/1 -> input summation/1(x1)
  leaky integration/1(Outport) -> piecewise lin./1
  input summation/1(out_1) -> leaky integration/1(Inport)
  Cortex/1 -> input summation/3(x3)

== system TRN_current/Basal Ganglia/STN/STN discrete model/2 input channel1 ==
  Salience : Inport  Orientation=down  Port=1  LatchInput=off
  GPe : Inport  Orientation=down  Port=2  LatchInput=off
  Cortex : Inport  Orientation=down  Port=3  LatchInput=off
  input summation : Subsystem  Orientation=down
  leaky integration : Subsystem  Orientation=down
  piecewise lin. : S-Function  Orientation=down  FunctionName=Mpieclin  Parameters=slope,thresh
  out : Outport  Orientation=down  InitialOutput=0
  wires:
  Cortex/1 -> input summation/3(x3)
  input summation/1(out_1) -> leaky integration/1(Inport)
  leaky integration/1(Outport) -> piecewise lin./1
  Salience/1 -> input summation/1(x1)
  GPe/1 -> input summation/2(x2)
  piecewise lin./1 -> out/1

== system TRN_current/Basal Ganglia/STN/STN discrete model/2 input channel2 ==
  Salience : Inport  Orientation=down  Port=1  LatchInput=off
  GPe : Inport  Orientation=down  Port=2  LatchInput=off
  Cortex : Inport  Orientation=down  Port=3  LatchInput=off
  input summation : Subsystem  Orientation=down
  leaky integration : Subsystem  Orientation=down
  piecewise lin. : S-Function  Orientation=down  FunctionName=Mpieclin  Parameters=slope,thresh
  out : Outport  Orientation=down  InitialOutput=0
  wires:
  piecewise lin./1 -> out/1
  GPe/1 -> input summation/2(x2)
  Salience/1 -> input summation/1(x1)
  leaky integration/1(Outport) -> piecewise lin./1
  input summation/1(out_1) -> leaky integration/1(Inport)
  Cortex/1 -> input summation/3(x3)

== system TRN_current/Basal Ganglia/STN/STN discrete model/2 input channel3 ==
  Salience : Inport  Orientation=down  Port=1  LatchInput=off
  GPe : Inport  Orientation=down  Port=2  LatchInput=off
  Cortex : Inport  Orientation=down  Port=3  LatchInput=off
  input summation : Subsystem  Orientation=down
  leaky integration : Subsystem  Orientation=down
  piecewise lin. : S-Function  Orientation=down  FunctionName=Mpieclin  Parameters=slope,thresh
  out : Outport  Orientation=down  InitialOutput=0
  wires:
  Cortex/1 -> input summation/3(x3)
  input summation/1(out_1) -> leaky integration/1(Inport)
  leaky integration/1(Outport) -> piecewise lin./1
  Salience/1 -> input summation/1(x1)
  GPe/1 -> input summation/2(x2)
  piecewise lin./1 -> out/1

== system TRN_current/Basal Ganglia/STN/STN discrete model/2 input channel4 ==
  Salience : Inport  Orientation=down  Port=1  LatchInput=off
  GPe : Inport  Orientation=down  Port=2  LatchInput=off
  Cortex : Inport  Orientation=down  Port=3  LatchInput=off
  input summation : Subsystem  Orientation=down
  leaky integration : Subsystem  Orientation=down
  piecewise lin. : S-Function  Orientation=down  FunctionName=Mpieclin  Parameters=slope,thresh
  out : Outport  Orientation=down  InitialOutput=0
  wires:
  piecewise lin./1 -> out/1
  GPe/1 -> input summation/2(x2)
  Salience/1 -> input summation/1(x1)
  leaky integration/1(Outport) -> piecewise lin./1
  input summation/1(out_1) -> leaky integration/1(Inport)
  Cortex/1 -> input summation/3(x3)

== system TRN_current/Basal Ganglia/STN/STN discrete model/2 input channel5 ==
  Salience : Inport  Orientation=down  Port=1  LatchInput=off
  GPe : Inport  Orientation=down  Port=2  LatchInput=off
  Cortex : Inport  Orientation=down  Port=3  LatchInput=off
  input summation : Subsystem  Orientation=down
  leaky integration : Subsystem  Orientation=down
  piecewise lin. : S-Function  Orientation=down  FunctionName=Mpieclin  Parameters=slope,thresh
  out : Outport  Orientation=down  InitialOutput=0
  wires:
  Cortex/1 -> input summation/3(x3)
  input summation/1(out_1) -> leaky integration/1(Inport)
  leaky integration/1(Outport) -> piecewise lin./1
  Salience/1 -> input summation/1(x1)
  GPe/1 -> input summation/2(x2)
  piecewise lin./1 -> out/1

== system TRN_current/Basal Ganglia/Striatum(D1)/chan1/leaky integration ==
  Inport : Inport  Port=1  PortDimensions=1  LatchInput=off
  Gain : Gain  Gain=A_rate  SaturateOnIntegerOverflow=on
  Integrator : Integrator
  decay const : Gain  Orientation=left  Gain=-A_rate  SaturateOnIntegerOverflow=on
  sum : Sum  SaturateOnIntegerOverflow=on  InputSameDT=on
  Outport : Outport  InitialOutput=0
  wires:
  decay const/1 -> sum/2
  sum/1 -> Integrator/1
  Integrator/1 -> decay const/1, Outport/1
  Inport/1 -> Gain/1
  Gain/1 -> sum/1

== system TRN_current/Basal Ganglia/Striatum(D1)/chan2/leaky integration ==
  Inport : Inport  Port=1  PortDimensions=1  LatchInput=off
  Gain : Gain  Gain=A_rate  SaturateOnIntegerOverflow=on
  Integrator : Integrator
  decay const : Gain  Orientation=left  Gain=-A_rate  SaturateOnIntegerOverflow=on
  sum : Sum  SaturateOnIntegerOverflow=on  InputSameDT=on
  Outport : Outport  InitialOutput=0
  wires:
  Gain/1 -> sum/1
  Inport/1 -> Gain/1
  Integrator/1 -> Outport/1, decay const/1
  sum/1 -> Integrator/1
  decay const/1 -> sum/2

== system TRN_current/Basal Ganglia/Striatum(D1)/chan3/leaky integration ==
  Inport : Inport  Port=1  PortDimensions=1  LatchInput=off
  Gain : Gain  Gain=A_rate  SaturateOnIntegerOverflow=on
  Integrator : Integrator
  decay const : Gain  Orientation=left  Gain=-A_rate  SaturateOnIntegerOverflow=on
  sum : Sum  SaturateOnIntegerOverflow=on  InputSameDT=on
  Outport : Outport  InitialOutput=0
  wires:
  decay const/1 -> sum/2
  sum/1 -> Integrator/1
  Integrator/1 -> decay const/1, Outport/1
  Inport/1 -> Gain/1
  Gain/1 -> sum/1

== system TRN_current/Basal Ganglia/Striatum(D1)/chan4/leaky integration ==
  Inport : Inport  Port=1  PortDimensions=1  LatchInput=off
  Gain : Gain  Gain=A_rate  SaturateOnIntegerOverflow=on
  Integrator : Integrator
  decay const : Gain  Orientation=left  Gain=-A_rate  SaturateOnIntegerOverflow=on
  sum : Sum  SaturateOnIntegerOverflow=on  InputSameDT=on
  Outport : Outport  InitialOutput=0
  wires:
  Gain/1 -> sum/1
  Inport/1 -> Gain/1
  Integrator/1 -> Outport/1, decay const/1
  sum/1 -> Integrator/1
  decay const/1 -> sum/2

== system TRN_current/Basal Ganglia/Striatum(D1)/chan5/leaky integration ==
  Inport : Inport  Port=1  PortDimensions=1  LatchInput=off
  Gain : Gain  Gain=A_rate  SaturateOnIntegerOverflow=on
  Integrator : Integrator
  decay const : Gain  Orientation=left  Gain=-A_rate  SaturateOnIntegerOverflow=on
  sum : Sum  SaturateOnIntegerOverflow=on  InputSameDT=on
  Outport : Outport  InitialOutput=0
  wires:
  decay const/1 -> sum/2
  sum/1 -> Integrator/1
  Integrator/1 -> decay const/1, Outport/1
  Inport/1 -> Gain/1
  Gain/1 -> sum/1

== system TRN_current/Basal Ganglia/Striatum(D1)/chan6/leaky integration ==
  Inport : Inport  Port=1  PortDimensions=1  LatchInput=off
  Gain : Gain  Gain=A_rate  SaturateOnIntegerOverflow=on
  Integrator : Integrator
  decay const : Gain  Orientation=left  Gain=-A_rate  SaturateOnIntegerOverflow=on
  sum : Sum  SaturateOnIntegerOverflow=on  InputSameDT=on
  Outport : Outport  InitialOutput=0
  wires:
  Gain/1 -> sum/1
  Inport/1 -> Gain/1
  Integrator/1 -> Outport/1, decay const/1
  sum/1 -> Integrator/1
  decay const/1 -> sum/2

== system TRN_current/Basal Ganglia/Striatum(D2)/chan1/leaky integration ==
  Inport : Inport  Port=1  PortDimensions=1  LatchInput=off
  Gain : Gain  Gain=A_rate  SaturateOnIntegerOverflow=on
  Integrator : Integrator
  decay const : Gain  Orientation=left  Gain=-A_rate  SaturateOnIntegerOverflow=on
  sum : Sum  SaturateOnIntegerOverflow=on  InputSameDT=on
  Outport : Outport  InitialOutput=0
  wires:
  Gain/1 -> sum/1
  Inport/1 -> Gain/1
  Integrator/1 -> Outport/1, decay const/1
  sum/1 -> Integrator/1
  decay const/1 -> sum/2

== system TRN_current/Basal Ganglia/Striatum(D2)/chan2/leaky integration ==
  Inport : Inport  Port=1  PortDimensions=1  LatchInput=off
  Gain : Gain  Gain=A_rate  SaturateOnIntegerOverflow=on
  Integrator : Integrator
  decay const : Gain  Orientation=left  Gain=-A_rate  SaturateOnIntegerOverflow=on
  sum : Sum  SaturateOnIntegerOverflow=on  InputSameDT=on
  Outport : Outport  InitialOutput=0
  wires:
  decay const/1 -> sum/2
  sum/1 -> Integrator/1
  Integrator/1 -> decay const/1, Outport/1
  Inport/1 -> Gain/1
  Gain/1 -> sum/1

== system TRN_current/Basal Ganglia/Striatum(D2)/chan3/leaky integration ==
  Inport : Inport  Port=1  PortDimensions=1  LatchInput=off
  Gain : Gain  Gain=A_rate  SaturateOnIntegerOverflow=on
  Integrator : Integrator
  decay const : Gain  Orientation=left  Gain=-A_rate  SaturateOnIntegerOverflow=on
  sum : Sum  SaturateOnIntegerOverflow=on  InputSameDT=on
  Outport : Outport  InitialOutput=0
  wires:
  Gain/1 -> sum/1
  Inport/1 -> Gain/1
  Integrator/1 -> Outport/1, decay const/1
  sum/1 -> Integrator/1
  decay const/1 -> sum/2

== system TRN_current/Basal Ganglia/Striatum(D2)/chan4/leaky integration ==
  Inport : Inport  Port=1  PortDimensions=1  LatchInput=off
  Gain : Gain  Gain=A_rate  SaturateOnIntegerOverflow=on
  Integrator : Integrator
  decay const : Gain  Orientation=left  Gain=-A_rate  SaturateOnIntegerOverflow=on
  sum : Sum  SaturateOnIntegerOverflow=on  InputSameDT=on
  Outport : Outport  InitialOutput=0
  wires:
  decay const/1 -> sum/2
  sum/1 -> Integrator/1
  Integrator/1 -> decay const/1, Outport/1
  Inport/1 -> Gain/1
  Gain/1 -> sum/1

== system TRN_current/Basal Ganglia/Striatum(D2)/chan5/leaky integration ==
  Inport : Inport  Port=1  PortDimensions=1  LatchInput=off
  Gain : Gain  Gain=A_rate  SaturateOnIntegerOverflow=on
  Integrator : Integrator
  decay const : Gain  Orientation=left  Gain=-A_rate  SaturateOnIntegerOverflow=on
  sum : Sum  SaturateOnIntegerOverflow=on  InputSameDT=on
  Outport : Outport  InitialOutput=0
  wires:
  Gain/1 -> sum/1
  Inport/1 -> Gain/1
  Integrator/1 -> Outport/1, decay const/1
  sum/1 -> Integrator/1
  decay const/1 -> sum/2

== system TRN_current/Basal Ganglia/Striatum(D2)/chan6/leaky integration ==
  Inport : Inport  Port=1  PortDimensions=1  LatchInput=off
  Gain : Gain  Gain=A_rate  SaturateOnIntegerOverflow=on
  Integrator : Integrator
  decay const : Gain  Orientation=left  Gain=-A_rate  SaturateOnIntegerOverflow=on
  sum : Sum  SaturateOnIntegerOverflow=on  InputSameDT=on
  Outport : Outport  InitialOutput=0
  wires:
  decay const/1 -> sum/2
  sum/1 -> Integrator/1
  Integrator/1 -> decay const/1, Outport/1
  Inport/1 -> Gain/1
  Gain/1 -> sum/1

== system TRN_current/Basal Ganglia/STN/STN discrete model/2 input channel/input summation ==
  x1 : Inport  Port=1  LatchInput=off
  x2 : Inport  Port=2  LatchInput=off
  x3 : Inport  Port=3  LatchInput=off
  Sum : Sum  Inputs=+++  SaturateOnIntegerOverflow=on  InputSameDT=on
  W1 : Gain  Gain=W_sal  SaturateOnIntegerOverflow=on
  W2 : Gain  Gain=W_GPe  SaturateOnIntegerOverflow=on
  W3 : Gain  Gain=W_Ctx  SaturateOnIntegerOverflow=on
  out_1 : Outport  InitialOutput=0
  wires:
  Sum/1 -> out_1/1
  x1/1 -> W1/1
  x2/1 -> W2/1
  W1/1 -> Sum/1
  W2/1 -> Sum/2
  x3/1 -> W3/1
  W3/1 -> Sum/3

== system TRN_current/Basal Ganglia/STN/STN discrete model/2 input channel/leaky integration ==
  Inport : Inport  Port=1  LatchInput=off
  Gain : Gain  Gain=A_rate  SaturateOnIntegerOverflow=on
  Integrator : Integrator
  decay const : Gain  Orientation=left  Gain=-A_rate  SaturateOnIntegerOverflow=on
  sum : Sum  SaturateOnIntegerOverflow=on  InputSameDT=on
  Outport : Outport  InitialOutput=0
  wires:
  decay const/1 -> sum/2
  sum/1 -> Integrator/1
  Integrator/1 -> Outport/1, decay const/1
  Inport/1 -> Gain/1
  Gain/1 -> sum/1

== system TRN_current/Basal Ganglia/STN/STN discrete model/2 input channel1/input summation ==
  x1 : Inport  Port=1  LatchInput=off
  x2 : Inport  Port=2  LatchInput=off
  x3 : Inport  Port=3  LatchInput=off
  Sum : Sum  Inputs=+++  SaturateOnIntegerOverflow=on  InputSameDT=on
  W1 : Gain  Gain=W_sal  SaturateOnIntegerOverflow=on
  W2 : Gain  Gain=W_GPe  SaturateOnIntegerOverflow=on
  W3 : Gain  Gain=W_Ctx  SaturateOnIntegerOverflow=on
  out_1 : Outport  InitialOutput=0
  wires:
  W3/1 -> Sum/3
  x3/1 -> W3/1
  W2/1 -> Sum/2
  W1/1 -> Sum/1
  x2/1 -> W2/1
  x1/1 -> W1/1
  Sum/1 -> out_1/1
